simulink model "untitled"  (R2020b)
settings: Solver=ode4  StartTime=0.0  StopTime=5  FixedStep=1e-3
values from neighbouring files (symbols this model uses):
  bm1 = 1.23e-05    [var.mat]    (also in var2.mat = 3.02e-06)
  bm2 = -3.45e-08    [var.mat]    (also in var2.mat = 1.63e-08)
  bp0 = 0.0014    [var.mat]    (also in var2.mat)
  bp1 = 0.001    [var.mat]    (also in var2.mat)
  g = 9.81    [var.mat]    (also in var2.mat)
  Jm = 1.2e-05    [var.mat]    (also in var2.mat = 8.62e-06)
  Jp = 0.00048    [var.mat]    (also in var2.mat)
  kaphi = 0.0157    [var.mat]    (also in var2.mat)
  ku1 = -8.98e-06    [var.mat]    (also in var2.mat = 5.38222507221e-05)
  ku2 = 3.18e-07    [var.mat]    (also in var2.mat = 3.49639864289e-07)
  ku3 = -2.45e-10    [var.mat]    (also in var2.mat = -7.23927342622e-10)
  ku4 = 3.90471830178e-13    [var2.mat]
  l = 0.068    [var.mat]    (also in var2.mat)
  La = 0.00868    [var.mat]    (also in var2.mat = 0.008673)
  m = 0.072    [var.mat]    (also in var2.mat)
  Ra = 12    [var.mat]    (also in var2.mat)
settings Model: Creator=Erick  LastModifiedBy=Erick

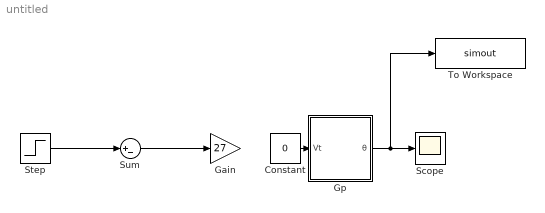
== system untitled ==
  Constant : Constant  Value=0
  Gain : Gain  Gain=27
  Gp : Subsystem
  Scope : Scope
  Step : Step  Time=0  After=50  SampleTime=0
  Sum : Sum  Inputs=|+-
  To Workspace : ToWorkspace  VariableName=simout  SaveFormat=Structure With Time  SampleTime=-1
  wires:
  Step/1 -> Sum/1
  Sum/1 -> Gain/1
  Constant/1 -> Gp/1(Vt)
  Gp/1(θ) -> To Workspace/1, Scope/1

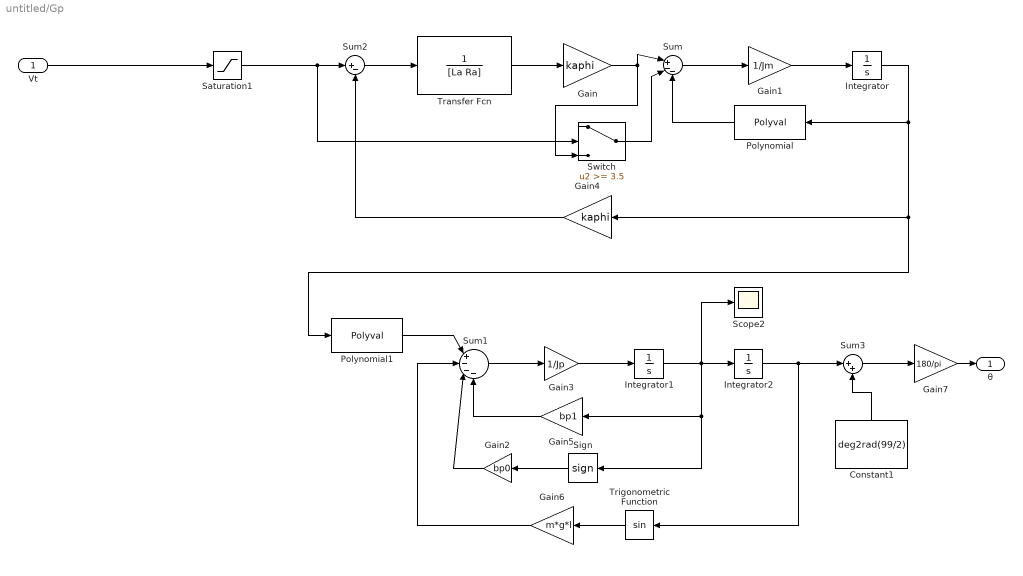
== system untitled/Gp ==
  Vt : Inport
  Constant1 : Constant  Value=deg2rad(99/2)
  Gain : Gain  Gain=kaphi
  Gain1 : Gain  Gain=1/Jm
  Gain2 : Gain  Gain=bp0
  Gain3 : Gain  Gain=1/Jp
  Gain4 : Gain  Gain=kaphi
  Gain5 : Gain  Gain=bp1
  Gain6 : Gain  Gain=m*g*l
  Gain7 : Gain  Gain=180/pi
  Integrator : Integrator
  Integrator1 : Integrator
  Integrator2 : Integrator  InitialCondition=deg2rad(99/2)  LimitOutput=on  UpperSaturationLimit=deg2rad(120)  LowerSaturationLimit=-deg2rad(120)
  Polynomial : Polyval  Coefs=[bm2, bm1, 0]
  Polynomial1 : Polyval  Coefs=[ku4, ku3, ku2, ku1, 0]
  Saturation1 : Saturate  UpperLimit=13.5  LowerLimit=0
  Scope2 : Scope
  Sign : Signum
  Sum : Sum  Inputs=|+--
  Sum1 : Sum  Inputs=|+---
  Sum2 : Sum  Inputs=|+-
  Sum3 : Sum  Inputs=|++
  Switch : Switch  Threshold=3.5
  Transfer Fcn : TransferFcn  Denominator=[La Ra]
  Trigonometric Function : Trigonometry
  θ : Outport
  wires:
  Transfer Fcn/1 -> Gain/1
  Polynomial/1 -> Sum/3
  Sum2/1 -> Transfer Fcn/1
  Gain4/1 -> Sum2/2
  Sum/1 -> Gain1/1
  Gain5/1 -> Sum1/4
  Gain/1 -> Switch/3, Sum/1
  Saturation1/1 -> Switch/2, Sum2/1
  Integrator1/1 -> Sign/1, Gain5/1, Scope2/1, Integrator2/1
  Switch/1 -> Sum/2
  Sum1/1 -> Gain3/1
  Gain1/1 -> Integrator/1
  Trigonometric Function/1 -> Gain6/1
  Integrator/1 -> Polynomial1/1, Gain4/1, Polynomial/1
  Gain6/1 -> Sum1/2
  Polynomial1/1 -> Sum1/1
  Gain3/1 -> Integrator1/1
  Gain2/1 -> Sum1/3
  Gain7/1 -> θ/1
  Vt/1 -> Saturation1/1
  Sign/1 -> Gain2/1
  Integrator2/1 -> Sum3/1, Trigonometric Function/1
  Sum3/1 -> Gain7/1
  Constant1/1 -> Sum3/2
